simulink model "adaptive_manipolatore"  (R2024b)
settings: Solver=VariableStepAuto  StartTime=0.0  StopTime=100  MaxStep=1e-5  RelTol=1e-3
values from neighbouring files (symbols this model uses):
  kd = K(:,3:4)    [regolatore_robot.m]
  kp = K(:,1:2)    [regolatore_robot.m]
  tau = 1    [regolatore_robot.m]
settings Model: Creator=Davide  LastModifiedBy=david
settings OptimizationCC: ReuseModelBlockBuffer=off
settings RTWCC: GPUComputeCapability=3.5

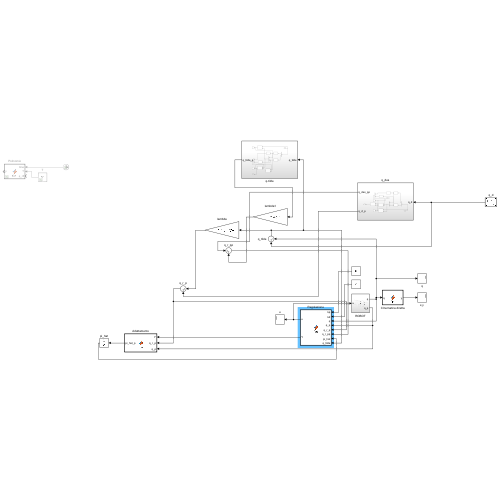
[thumbnail: Simulink's stored preview of the top-level diagram]
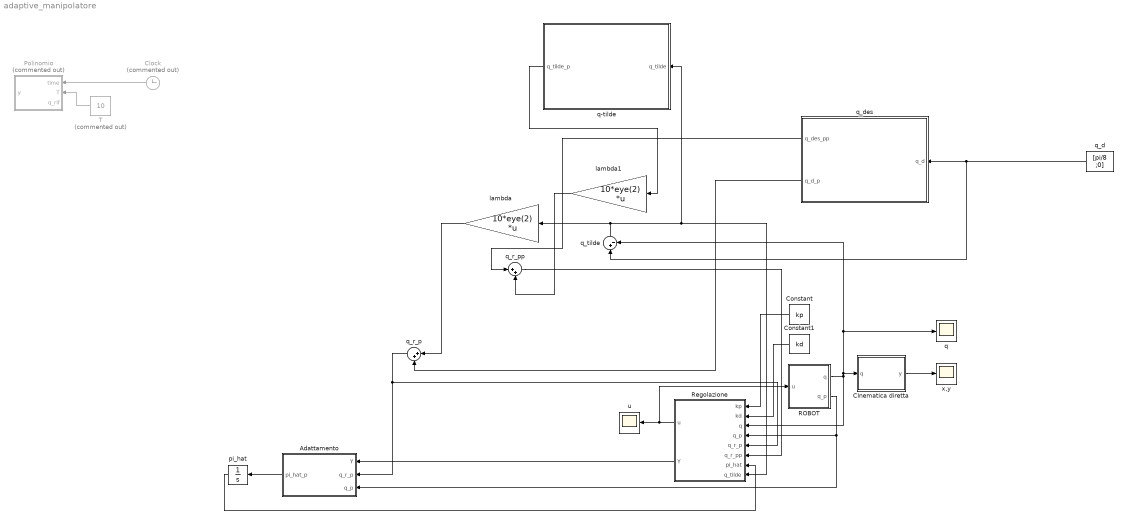
== system adaptive_manipolatore ==
  Adattamento : MATLAB Function  TreatAsAtomicUnit=on
  CInematica diretta : MATLAB Function  TreatAsAtomicUnit=on
  Clock : Clock  Commented=on
  Constant : Constant  Value=kp  VectorParams1D=off
  Constant1 : Constant  Value=kd  VectorParams1D=off
  Polinomio : MATLAB Function  Commented=on  TreatAsAtomicUnit=on
  ROBOT : Subsystem
  Regolazione : MATLAB Function  TreatAsAtomicUnit=on
  T : Constant  Commented=on  Value=10  VectorParams1D=off
  lambda : Gain  Gain=10*eye(2)  Multiplication=Matrix(K*u)
  lambda1 : Gain  Gain=10*eye(2)  Multiplication=Matrix(K*u)
  pi_hat : Integrator  InitialCondition=zeros(7,1)
  q : Scope
  q-tilde : Subsystem
  q_d : Constant  Value=[pi/8 ;0]  VectorParams1D=off
  q_des : Subsystem
  q_r_p : Sum  Inputs=|++
  q_r_pp : Sum  Inputs=|++
  q_tilde : Sum  Inputs=|+-
  u : Scope
  x,y : Scope
  wires:
  Adattamento/1(pi_hat_p) -> pi_hat/1
  T/1 -> Polinomio/2(T)
  ROBOT/2(q_p) -> Regolazione/4(q_p), Adattamento/3(q_p)
  Clock/1 -> Polinomio/1(time)
  q_r_p/1 -> Adattamento/2(q_r_p), Regolazione/5(q_r_p)
  ROBOT/1(q) -> CInematica diretta/1(q), q/1, q_tilde/2, Regolazione/3(q)
  lambda/1 -> q_r_p/1
  q_r_pp/1 -> Regolazione/6(q_r_pp)
  lambda1/1 -> q_r_pp/2
  q_tilde/1 -> q-tilde/1(q_tilde), Regolazione/8(q_tilde), lambda/1
  Regolazione/2(Y) -> Adattamento/1(Y)
  Regolazione/1(u) -> ROBOT/1(u), u/1
  Constant1/1 -> Regolazione/2(kd)
  q_d/1 -> q_des/1(q_d), q_tilde/1
  CInematica diretta/1(y) -> x,y/1
  q_des/1(q_des_pp) -> q_r_pp/1
  q_des/2(q_d_p) -> q_r_p/2
  q-tilde/1(q_tilde_p) -> lambda1/1
  Constant/1 -> Regolazione/1(kp)
  pi_hat/1 -> Regolazione/7(pi_hat)

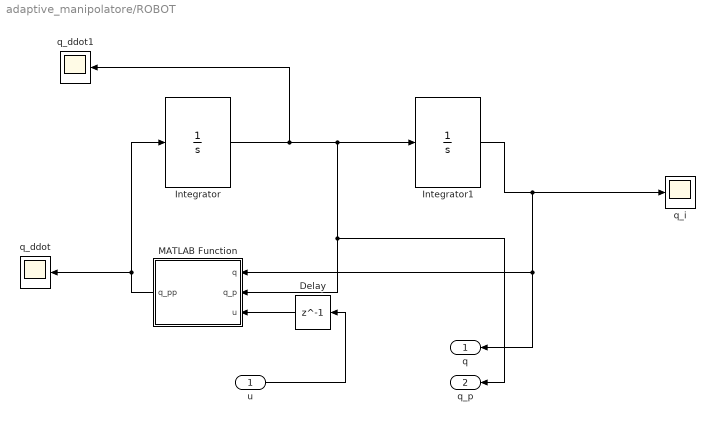
== system adaptive_manipolatore/ROBOT ==
  u : Inport  PortDimensions=[2,1]
  Delay : Delay  DelayLength=1  InitialCondition=0
  Integrator : Integrator  InitialCondition=[0 ; 0]  ZeroCross=off
  Integrator1 : Integrator  InitialCondition=[0 ; 0]  ZeroCross=off
  MATLAB Function : MATLAB Function  TreatAsAtomicUnit=on
  q_ddot : Scope
  q_ddot1 : Scope
  q_i : Scope
  q : Outport  PortDimensions=[2,1]
  q_p : Outport  Port=2  PortDimensions=[2,1]
  wires:
  Integrator/1 -> q_ddot1/1, q_p/1, MATLAB Function/2(q_p), Integrator1/1
  MATLAB Function/1(q_pp) -> Integrator/1, q_ddot/1
  Integrator1/1 -> q/1, MATLAB Function/1(q), q_i/1
  u/1 -> Delay/1
  Delay/1 -> MATLAB Function/3(u)

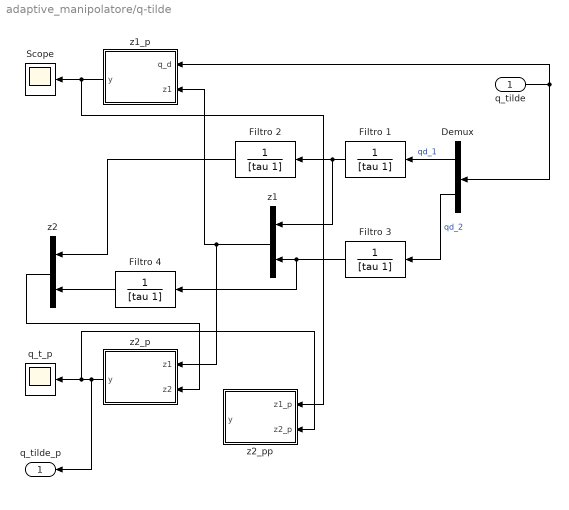
== system adaptive_manipolatore/q-tilde ==
  q_tilde : Inport
  Demux : Demux  Outputs=2
  Filtro {1..4} (4 alike) : TransferFcn  Denominator=[tau 1]
  Scope : Scope
  q_t_p : Scope
  z1 : Mux  Inputs=2
  z1_p : MATLAB Function  TreatAsAtomicUnit=on
  z2 : Mux  Inputs=2
  z2_p : MATLAB Function  TreatAsAtomicUnit=on
  z2_pp : MATLAB Function  TreatAsAtomicUnit=on
  q_tilde_p : Outport
  wires:
  z2/1 -> z2_p/2(z2)
  Filtro 3/1 -> z1/2, Filtro 4/1
  z1_p/1(y) -> Scope/1, z2_pp/1(z1_p)
  Filtro 1/1 -> Filtro 2/1, z1/1
  Filtro 2/1 -> z2/1
  Filtro 4/1 -> z2/2
  z1/1 -> z2_p/1(z1), z1_p/2(z1)
  z2_p/1(y) -> q_t_p/1, z2_pp/2(z2_p), q_tilde_p/1
  Demux/2 -> Filtro 3/1  "qd_2"
  Demux/1 -> Filtro 1/1  "qd_1"
  q_tilde/1 -> Demux/1, z1_p/1(q_d)

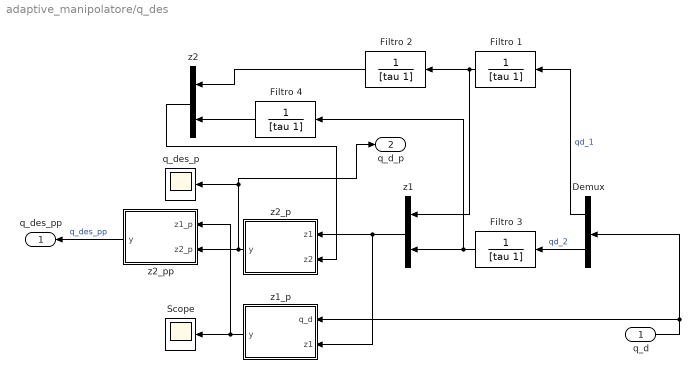
== system adaptive_manipolatore/q_des ==
  q_d : Inport
  Demux : Demux  Outputs=2
  Filtro {1..4} (4 alike) : TransferFcn  Denominator=[tau 1]
  Scope : Scope
  q_des_p : Scope
  z1 : Mux  Inputs=2
  z1_p : MATLAB Function  TreatAsAtomicUnit=on
  z2 : Mux  Inputs=2
  z2_p : MATLAB Function  TreatAsAtomicUnit=on
  z2_pp : MATLAB Function  TreatAsAtomicUnit=on
  q_des_pp : Outport
  q_d_p : Outport  Port=2
  wires:
  z2_p/1(y) -> q_d_p/1, q_des_p/1, z2_pp/2(z2_p)
  z2/1 -> z2_p/2(z2)
  z2_pp/1(y) -> q_des_pp/1  "q_des_pp"
  Filtro 1/1 -> z1/1, Filtro 2/1
  Filtro 2/1 -> z2/1
  Filtro 4/1 -> z2/2
  z1/1 -> z2_p/1(z1), z1_p/2(z1)
  z1_p/1(y) -> z2_pp/1(z1_p), Scope/1
  Filtro 3/1 -> Filtro 4/1, z1/2
  Demux/2 -> Filtro 3/1  "qd_2"
  Demux/1 -> Filtro 1/1  "qd_1"
  q_d/1 -> z1_p/1(q_d), Demux/1

== matlab function adaptive_manipolatore/q-tilde/z2_p ==
  data: z1 input; z2 input; y output
function y = fcn(z1,z2)


tau = 1;
z2_p = (-1/tau)*z2+z1;

y = z2_p;

== matlab function adaptive_manipolatore/q-tilde/z2_pp ==
  data: z1_p input; z2_p input; y output
function y = fcn(z1_p,z2_p)



tau = 1;
z2_pp = (-1/tau)*z2_p+z1_p;

y = z2_pp;

== matlab function adaptive_manipolatore/ROBOT/MATLAB Function ==
  data: q input; q_p input; u input; q_pp output
function q_pp = fcn(q,q_p,u)


theta1 = 10.6125; 
theta2 = 0.85; 
theta3 = 2.25;
theta4 = 1.6;
theta5 = 80.9325;
theta6 = 14.7150;
%q = q_i;
%q_p = q_p_i;
%v = u;
F1 = 15;
F2 = 10;

B = [theta1 + 2*theta3*q(2) theta2+theta3*cos(q(2)) ; ...
     theta2+theta3*cos(q(2)) theta4];
C = [-2*theta3*q_p(2)*sin(q(2))  -theta3*q_p(2)*sin(q(2)) ; ...
      theta3*q_p(1)*sin(q(2))              0              ];
g = [theta5*cos(q(1))+theta6*cos(q(1)+q(2)) ; theta6*cos(q(1)+q(2))];
F = [F1*q_p(1) ; F2*q_p(2)];

q_pp = inv(B)*(u - g - F - C*q_p);

== matlab function adaptive_manipolatore/Regolazione ==
  data: kp input; kd input; q input size=[2,1]; q_p input size=[2,1]; q_r_p input; q_r_pp input; u output size=[2,1]; pi_hat input size=[7,1]; Y output size=[2,7]; q_tilde input
function [u,Y] = fcn(kp,kd,q,q_p,q_r_p,q_r_pp,pi_hat,q_tilde)


%Calcolo di sigma 
sigma = q_r_p - q_p;

% Costruzione della matrice di regressore Y
Y1 = [q_r_pp(1) , q_r_pp(2) , 2*cos(q(2))*q_r_pp(1)+cos(q(2))*q_r_pp(2)-sin(q(2))*(q_p(2)^2), cos(q(1)), cos(q(1)+q(2)), q_p(1) , 0];
Y2 = [0 , q_r_pp(2) , cos(q(2))*q_r_pp(1)+sin(q(2))*(q_p(1)^2), 0, cos(q(1)+q(2)), 0 , q_p(2)];

%Output
Y = [Y1;Y2];
u = Y*pi_hat + kd*sigma + kp*q_tilde;

== matlab function adaptive_manipolatore/Polinomio ==
  data: time input; T input; q_rif input; y output
function y = fcn(time,T,q_rif)



% q_r = q_rif;
% a3 = (-2*q_r)/t;
% a2 = (3*q_r)/t;
% a1 = [0;0];
% a0 = [0;0];
% p_t = a3*time^3+a2*time^2+a1*time+a0;


% Condizioni iniziali e finali per q_r1
q1_init = 0; % Posizione iniziale per q_r1
q1_final = pi/8; % Posizione finale per q_r1

% Condizioni iniziali e finali per q_r2
q2_init = 0; % Posizione iniziale per q_r2
q2_final = pi/8; % Posizione finale per q_r2

% Sistema di equazioni per i coefficienti di q_r1
A = [0,     0,     0,     1;   % q_r1(0) = a0
     T^3,   T^2,   T,     1;   % q_r1(T) = a3*T^3 + a2*T^2 + a1*T + a0
     0,     0,     1,     0;   % dq_r1/dt(0) = a1
     3*T^2, 2*T,   1,     0];  % dq_r1/dt(T) = 3*a3*T^2 + 2*a2*T + a1

b1 = [q1_init; q1_final; 0; 0]; % Vettore delle condizioni al contorno per q_r1
b2 = [q2_init; q2_final; 0; 0]; % Vettore delle condizioni al contorno per q_r2

% Risoluzione del sistema lineare per q_r1 e q_r2
coefficients1 = A \ b1; % Coefficienti per q_r1
coefficients2 = A \ b2; % Coefficienti per q_r2

% Assegnazione dei coefficienti per q_r1
a31 = coefficients1(1);
a21 = coefficients1(2);
a11 = coefficients1(3);
a01 = coefficients1(4);

% Assegnazione dei coefficienti per q_r2
a32 = coefficients2(1);
a22 = coefficients2(2);
a12 = coefficients2(3);
a02 = coefficients2(4);

% Definizione dei polinomi
q_r1 = a31 * time^3 + a21 * time^2 + a11 * time + a01; % Polinomio per q_r1
q_r2 = a32 * time^3 + a22 * time^2 + a12 * time + a02; % Polinomio per q_r2

p_t = [q_r1 ; q_r2];

y = p_t;

== matlab function adaptive_manipolatore/CInematica diretta ==
  data: q input; y output
function y = fcn(q)

l1 = 1.5;
l2 = 1;

%Estrazione posizione spazio operativo
y = [l1*cos(q(1))+l2*cos(q(2)) ; l1*sin(q(1))+l2*sin(q(2))];

== matlab function adaptive_manipolatore/q_des/z1_p ==
  data: q_d input; z1 input; y output
function y = fcn(q_d,z1)


q = q_d;
tau = 1;
z1_p = (-1/tau)*z1+q;

y = z1_p;

== matlab function adaptive_manipolatore/q_des/z2_p ==
  data: z1 input; z2 input; y output
function y = fcn(z1,z2)


tau = 1;
z2_p = (-1/tau)*z2+z1;

y = z2_p;

== matlab function adaptive_manipolatore/q_des/z2_pp ==
  data: z1_p input; z2_p input; y output
function y = fcn(z1_p,z2_p)



tau = 1;
z2_pp = (-1/tau)*z2_p+z1_p;

y = z2_pp;

== matlab function adaptive_manipolatore/Adattamento ==
  data: Y input; pi_hat_p output; q_r_p input; q_p input
function pi_hat_p = fcn(Y,q_r_p,q_p)

K_i = 1*eye(7);
sigma = q_r_p - q_p;
pi_hat_p = inv(K_i)*Y'*sigma;

== matlab function adaptive_manipolatore/q-tilde/z1_p ==
  data: q_d input; z1 input; y output
function y = fcn(q_d,z1)


q = q_d;
tau = 1;
z1_p = (-1/tau)*z1+q;

y = z1_p;
